simulink model "sepicmm_vs_sepicsm_1"  (R2015a)
settings: Solver=ode45  StartTime=0.0  StopTime=1  RelTol=1e-3
values from neighbouring files (symbols this model uses):
  alpha = min(d1,d2)    [Final_2.m]    (also in Final_discreto.m)
  C = [0 0 0 1]    [Final_2.m]    (also in Final_discreto.m)
  C1 = 190e-6    (= 0.00019)    [Final_2.m]    (also in Final_discreto.m = 0.0022)
  C2 = 190e-6    (= 0.00019)    [Final_2.m]    (also in Final_discreto.m = 0.0022)
  E0 = 20    [Final_2.m]    (also in Final_discreto.m = 36)
  L = L'    [Final_2.m]
  L1 = 2.3e-3    (= 0.0023)    [Final_2.m]    (also in Final_discreto.m = 0.00156)
  L2 = 330e-6    (= 0.00033)    [Final_2.m]    (also in Final_discreto.m = 0.00324)
  R0 = 44    [Final_2.m]    (also in Final_discreto.m = 50)
  R1 = 2.134    [Final_2.m]    (also in Final_discreto.m = 0.3)
  R2 = 0.234    [Final_2.m]    (also in Final_discreto.m = 0.3)
  V0 = 20    [Final_2.m]    (also in Final_discreto.m = 120)
undefined symbols (not defined in the file or in its folder): Rl
libraries: powerlib x28, powerlib_meascontrol x1
settings Model: Creator=berme_000  LastModifiedBy=berme_000

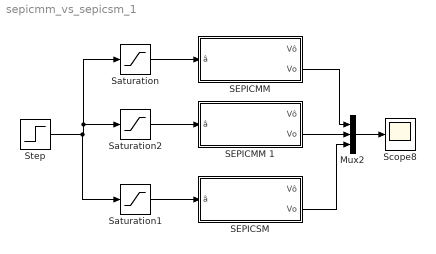
== system sepicmm_vs_sepicsm_1 ==
  Mux2 : Mux  Inputs=3
  "SEPICMM " : Subsystem
  SEPICMM 1 : Subsystem
  "SEPICSM " : Subsystem
  Saturation : Saturate  UpperLimit=1  LowerLimit=0
  Saturation1 : Saturate  UpperLimit=1  LowerLimit=0
  Saturation2 : Saturate  UpperLimit=1  LowerLimit=0
  Scope8 : Scope
      settings: YMin=-60  YMax=130  SaveName=ScopeData9
  Step : Step  Time=0.5  After=alpha  SampleTime=0
  wires:
  Saturation/1 -> "SEPICMM "/1(â)
  Saturation1/1 -> "SEPICSM "/1(â)
  Mux2/1 -> Scope8/1
  "SEPICMM "/2(Vo) -> Mux2/1
  "SEPICSM "/2(Vo) -> Mux2/3
  Step/1 -> Saturation1/1, Saturation2/1, Saturation/1
  Saturation2/1 -> SEPICMM 1/1(â)
  SEPICMM 1/2(Vo) -> Mux2/2

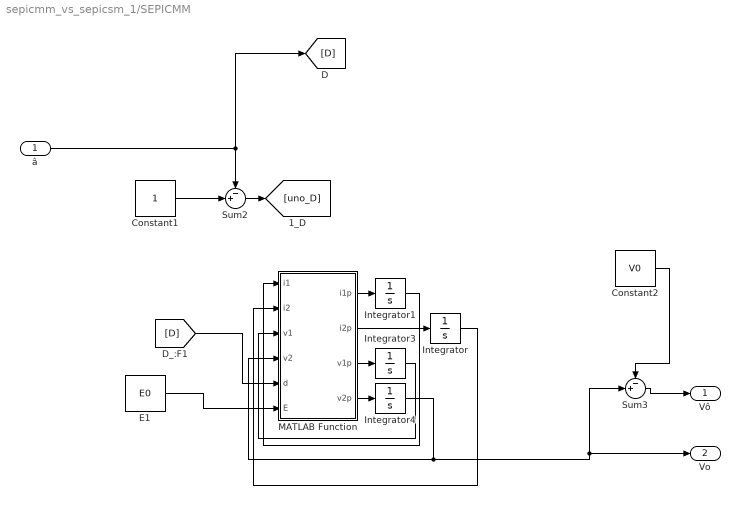
== system sepicmm_vs_sepicsm_1/SEPICMM  ==
  â : Inport
  Constant1 : Constant
  Constant2 : Constant  Value=V0
  E1 : Constant  Value=E0
  Integrator{,1,3..4} (4 alike) : Integrator
  MATLAB Function : MATLAB Function  TreatAsAtomicUnit=on
  Sum2 : Sum  Inputs=-+|
  Sum3 : Sum  Inputs=-+|
  Vô : Outport
  Vo : Outport  Port=2
  wires:
  â/1 -> [D], Sum2/1
  Constant1/1 -> Sum2/2
  Constant2/1 -> Sum3/1
  Sum3/1 -> Vô/1
  Sum2/1 -> [uno_D]
  E1/1 -> MATLAB Function/6(E)
  [D] -> MATLAB Function/5(d)
  MATLAB Function/2(i2p) -> Integrator/1
  MATLAB Function/1(i1p) -> Integrator1/1
  MATLAB Function/4(v2p) -> Integrator4/1
  MATLAB Function/3(v1p) -> Integrator3/1
  Integrator1/1 -> MATLAB Function/1(i1)
  Integrator/1 -> MATLAB Function/2(i2)
  Integrator3/1 -> MATLAB Function/3(v1)
  Integrator4/1 -> Sum3/2, Vo/1, MATLAB Function/4(v2)

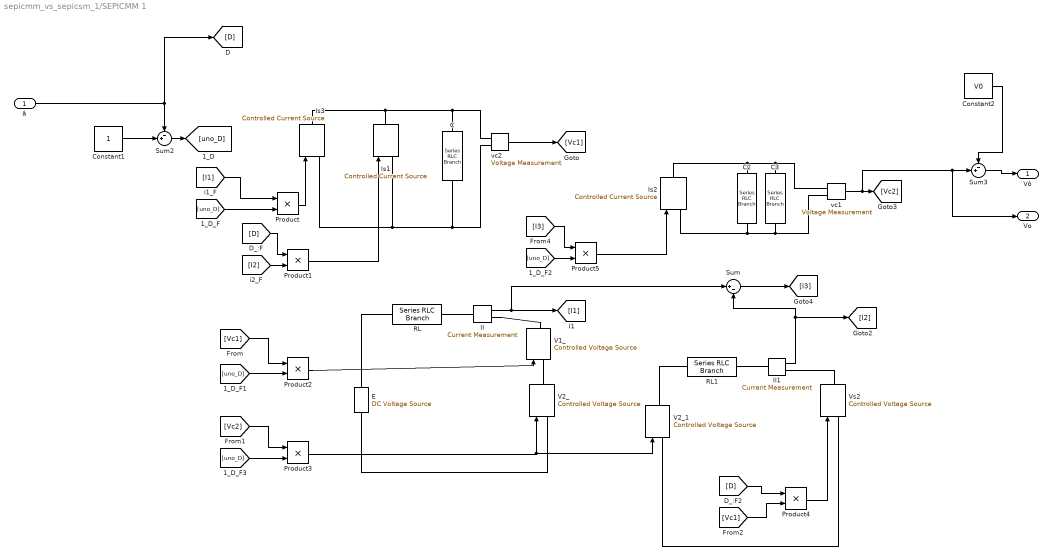
== system sepicmm_vs_sepicsm_1/SEPICMM 1 ==
  â : Inport
  C : powerlib/Elements/Series RLC Branch  LConnTagsString=__new0  RConnTagsString=__new0  BranchType=C  Resistance=Rl  Inductance=L  SetiL0=off  InitialCurrent=0  Capacitance=C1  Setx0=off  InitialVoltage=Vc1  Measurements=None
  C2 : powerlib/Elements/Series RLC Branch  LConnTagsString=__new0  RConnTagsString=__new0  BranchType=C  Resistance=Rl  Inductance=L  SetiL0=off  InitialCurrent=0  Capacitance=C2  Setx0=off  InitialVoltage=V0  Measurements=None
  C3 : powerlib/Elements/Series RLC Branch  LConnTagsString=__new0  RConnTagsString=__new0  BranchType=R  Resistance=R0  Inductance=L  SetiL0=off  InitialCurrent=0  Capacitance=C  Setx0=off  InitialVoltage=0  Measurements=None
  Constant1 : Constant
  Constant2 : Constant  Value=V0
  E : powerlib/Electrical Sources/DC Voltage Source  Amplitude=E0  Measurements=Voltage
  Il : powerlib/Measurements/Current Measurement  PhasorSimulation=off  OutputType=Complex  PSBequivalent=0
  Il1 : powerlib/Measurements/Current Measurement  PhasorSimulation=off  OutputType=Complex  PSBequivalent=0
  Is1 : powerlib/Electrical Sources/Controlled Current Source  Initialize=on  Source_Type=AC  Amplitude=0  Phase=0  Frequency=0  Measurements=None
  Is2 : powerlib/Electrical Sources/Controlled Current Source  Initialize=on  Source_Type=AC  Amplitude=0  Phase=0  Frequency=0  Measurements=None
  Is3 : powerlib/Electrical Sources/Controlled Current Source  Initialize=on  Source_Type=AC  Amplitude=0  Phase=0  Frequency=0  Measurements=None
  Product{,1..5} (6 alike) : Product
  RL : powerlib/Elements/Series RLC Branch  LConnTagsString=__new0  RConnTagsString=__new0  BranchType=RL  Resistance=R1  Inductance=L1  SetiL0=off  InitialCurrent=il1  Capacitance=1e-6  Setx0=off  InitialVoltage=0  Measurements=None
  RL1 : powerlib/Elements/Series RLC Branch  LConnTagsString=__new0  RConnTagsString=__new0  BranchType=RL  Resistance=R2  Inductance=L2  SetiL0=off  InitialCurrent=il2  Capacitance=1e-6  Setx0=off  InitialVoltage=0  Measurements=None
  Sum : Sum  Inputs=|+-
  Sum2 : Sum  Inputs=-+|
  Sum3 : Sum  Inputs=-+|
  V1_ : powerlib/Electrical Sources/Controlled Voltage Source  Initialize=on  Source_Type=AC  Amplitude=0  Phase=0  Frequency=0  Measurements=None
  V2_ : powerlib/Electrical Sources/Controlled Voltage Source  Initialize=on  Source_Type=AC  Amplitude=0  Phase=0  Frequency=0  Measurements=None
  V2_1 : powerlib/Electrical Sources/Controlled Voltage Source  Initialize=on  Source_Type=AC  Amplitude=0  Phase=0  Frequency=0  Measurements=None
  Vs2 : powerlib/Electrical Sources/Controlled Voltage Source  Initialize=on  Source_Type=AC  Amplitude=0  Phase=0  Frequency=0  Measurements=None
  vc1 : powerlib/Measurements/Voltage Measurement  PhasorSimulation=off  OutputType=Complex  PSBequivalent=0
  vc2 : powerlib/Measurements/Voltage Measurement  PhasorSimulation=off  OutputType=Complex  PSBequivalent=0
  Vô : Outport
  Vo : Outport  Port=2
  wires:
  Il/1 -> Sum/1, [I1]
  Il1/1 -> [I2], Sum/2
  vc2/1 -> [Vc1]
  Sum/1 -> [I3]
  â/1 -> [D], Sum2/1
  Constant1/1 -> Sum2/2
  Constant2/1 -> Sum3/1
  vc1/1 -> Vo/1, Sum3/2, [Vc2]
  Sum3/1 -> Vô/1
  [I1] -> Product/1
  Product/1 -> Is3/1
  [uno_D] -> Product/2
  [I2] -> Product1/2
  [D] -> Product1/1
  Product1/1 -> Is1/1
  [uno_D] -> Product2/2
  [Vc1] -> Product2/1
  Product2/1 -> V1_/1
  [Vc2] -> Product3/1
  [uno_D] -> Product3/2
  Product3/1 -> V2_/1, V2_1/1
  Product4/1 -> Vs2/1
  [Vc1] -> Product4/2
  [uno_D] -> Product5/2
  [I3] -> Product5/1
  Product5/1 -> Is2/1
  Sum2/1 -> [uno_D]
  [D] -> Product4/1
  connections:
  V2_/RConn1 -- V1_/LConn1
  V2_/LConn1 -- E/LConn1
  C/RConn1 -- Is3/LConn1 -- Is1/LConn1 -- vc2/LConn2
  C2/LConn1 -- Is2/RConn1 -- vc1/LConn1 -- C3/LConn1
  Is2/LConn1 -- C2/RConn1 -- vc1/LConn2 -- C3/RConn1
  Is3/RConn1 -- Is1/RConn1 -- C/LConn1 -- vc2/LConn1
  Il/RConn1 -- V1_/RConn1
  RL/LConn1 -- E/RConn1
  Il/LConn1 -- RL/RConn1
  Il1/LConn1 -- RL1/RConn1
  Il1/RConn1 -- Vs2/RConn1
  V2_1/RConn1 -- RL1/LConn1
  V2_1/LConn1 -- Vs2/LConn1

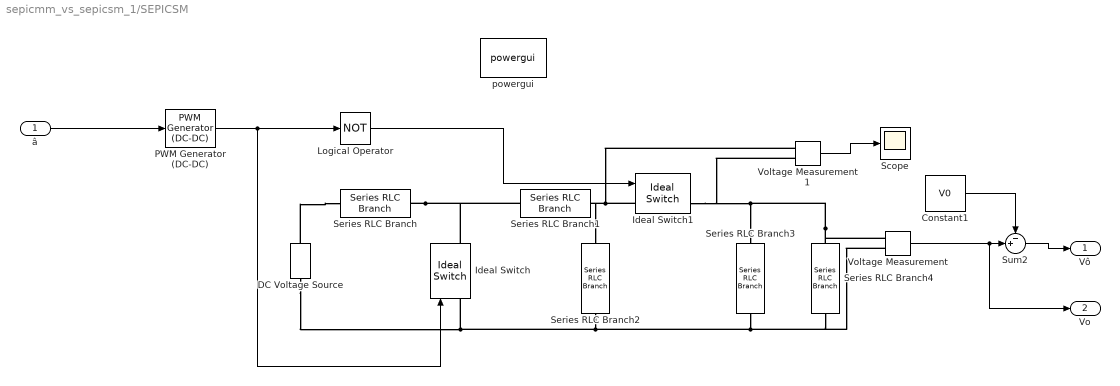
== system sepicmm_vs_sepicsm_1/SEPICSM  ==
  â : Inport
  Constant1 : Constant  Value=V0
  DC Voltage Source : powerlib/Electrical Sources/DC Voltage Source  Amplitude=E0  Measurements=None
  Ideal Switch : powerlib/Power Electronics/Ideal Switch  Ron=0.001  Lon=0  IC=0  Rs=1e5  Cs=inf  Measurements=on
  Ideal Switch1 : powerlib/Power Electronics/Ideal Switch  Ron=0.001  Lon=0  IC=0  Rs=1e5  Cs=inf  Measurements=on
  Logical Operator : Logic  Operator=NOT  AllPortsSameDT=off  OutDataTypeStr=boolean
  PWM Generator (DC-DC) : powerlib_meascontrol/Pulse & Signal Generators/PWM Generator (DC-DC)  Fsw=50000  Ts=0
  Scope : Scope
      settings: YMin=-9.23568e-13  YMax=-9.23568e-13  SaveName=ScopeData2
  Series RLC Branch : powerlib/Elements/Series RLC Branch  LConnTagsString=__new0  RConnTagsString=__new0  BranchType=RL  Resistance=R1  Inductance=L1  SetiL0=on  InitialCurrent=0  Capacitance=1e-6  Setx0=off  InitialVoltage=0  Measurements=None
  Series RLC Branch1 : powerlib/Elements/Series RLC Branch  LConnTagsString=__new0  RConnTagsString=__new0  BranchType=C  Resistance=1  Inductance=L1  SetiL0=off  InitialCurrent=0  Capacitance=C1  Setx0=on  InitialVoltage=0  Measurements=None
  Series RLC Branch2 : powerlib/Elements/Series RLC Branch  LConnTagsString=__new0  RConnTagsString=__new0  BranchType=RL  Resistance=R2  Inductance=L2  SetiL0=on  InitialCurrent=0  Capacitance=1e-6  Setx0=off  InitialVoltage=0  Measurements=None
  Series RLC Branch3 : powerlib/Elements/Series RLC Branch  LConnTagsString=__new0  RConnTagsString=__new0  BranchType=C  Resistance=1  Inductance=L1  SetiL0=off  InitialCurrent=0  Capacitance=C2  Setx0=on  InitialVoltage=0  Measurements=None
  Series RLC Branch4 : powerlib/Elements/Series RLC Branch  LConnTagsString=__new0  RConnTagsString=__new0  BranchType=R  Resistance=R0  Inductance=L1  SetiL0=off  InitialCurrent=0  Capacitance=1e-6  Setx0=off  InitialVoltage=0  Measurements=None
  Sum2 : Sum  Inputs=-+|
  Voltage Measurement : powerlib/Measurements/Voltage Measurement  PhasorSimulation=off  OutputType=Complex  PSBequivalent=0
  Voltage Measurement1 : powerlib/Measurements/Voltage Measurement  PhasorSimulation=off  OutputType=Complex  PSBequivalent=0
  powergui : powerlib/powergui  Priority=1  SimulationMode=Continuous  SolverType=Tustin  SampleTime=50e-6  frequency=60  SPID=off  DisableSnubberDevices=off  DisableRonSwitches=off  DisableVfSwitches=off  SwTol=0  DisplayEquations=off  Interpol=off  methode=off  Ts=0  FunctionMessages=off  echomessages=off  HookPort=off  EnableUseOfTLC=off  x0status=blocks  frequencyindice=0  Pbase=100e6  ErrMax=1e-4  Iterations=50  UnitsV=kV  UnitsW=MW  buscounter=0  RestoreLinks=warning  ResistiveCurrentMeasurement=off  Frange=[0:2:500]  Ylog=off  Xlog=on  ShowGrid=off  save=off  variable=ZData  structure=0  ZoomFFT=off  StartTime=0.0  cycles=1  DisplayStyle=1  fundamental=60  FreqAxis=off  MaxFrequency=1000  frequencyindicesteady=1  RmsSteady=1  display=off
  Vô : Outport
  Vo : Outport  Port=2
  wires:
  â/1 -> PWM Generator (DC-DC)/1
  PWM Generator (DC-DC)/1 -> Logical Operator/1, Ideal Switch/1
  Logical Operator/1 -> Ideal Switch1/1
  Voltage Measurement1/1 -> Scope/1
  Constant1/1 -> Sum2/1
  Voltage Measurement/1 -> Vo/1, Sum2/2
  Sum2/1 -> Vô/1
  connections:
  Series RLC Branch/RConn1 -- Series RLC Branch1/LConn1 -- Ideal Switch/RConn1
  Ideal Switch1/LConn1 -- Series RLC Branch1/RConn1 -- Series RLC Branch2/RConn1 -- Voltage Measurement1/LConn1
  Series RLC Branch2/LConn1 -- DC Voltage Source/LConn1 -- Ideal Switch/LConn1 -- Series RLC Branch3/RConn1 -- Voltage Measurement/LConn2 -- Series RLC Branch4/RConn1
  Voltage Measurement/LConn1 -- Series RLC Branch4/LConn1 -- Series RLC Branch3/LConn1 -- Ideal Switch1/RConn1 -- Voltage Measurement1/LConn2
  DC Voltage Source/RConn1 -- Series RLC Branch/LConn1

== matlab function sepicmm_vs_sepicsm_1/SEPICMM /MATLAB Function ==
  data: i1 input; i2 input; v1 input; v2 input; i1p output; d input; E input; i2p output; v1p output; v2p output
function [i1p,i2p,v1p,v2p]  = fcn(i1,i2,v1,v2,d,E)
%#codegen
l1=1.56e-3;
l2=3.24e-3;
r0=50;
r1=0.3;
r2=0.3;
c1=2.2e-3;
c2=2.2e-3;
i1p=(E-i1*r1-(1-d)*(v1+v2))/l1;
i2p=(-v1*d+(1-d)*v2-i2*r2)/l2;
v1p=(i2*d+i1*(1-d))/c1;
v2p=(-v2/r0+(1-d)*(i1-i2))/c2;
